simulink model "EMJ1"  (R2022b)
settings: Solver=VariableStepAuto  StartTime=0.0  StopTime=sim_time  FixedStep=0.001  RelTol=1e-3
values from neighbouring files (symbols this model uses):
  alpha = 0    [PMS.m]
  B = 0.24    [PMS.m]
  i = i:0.05:(i+0.5)    [PMS.m]
  Kb = 0.35    [PMS.m]
  Kt = 0.9    [PMS.m]
  L = 2.5  * (10^-3)    (= 0.0025)    [PMS.m]
  R = 0.03    [PMS.m]
  r = 0.3    [PMS.m]
  slope = 1    [PMS.m]
  v = 0    [PMS.m]
  velocity = 1    [PMS.m]
  W = 45    [PMS.m]
  X = 0.46    [PMS.m]
  Y = 300    [PMS.m]
  Z = 3000    [PMS.m]
libraries: simulink x1
settings Model: Creator=Gebruiker  LastModifiedBy=Gebruiker
settings SolverCC: MaxConsecutiveMinStep=2
settings DataIOCC: ReturnWorkspaceOutputs=off
settings ModelReferenceCC: EnableRefExpFcnMdlSchedulingChecks=on

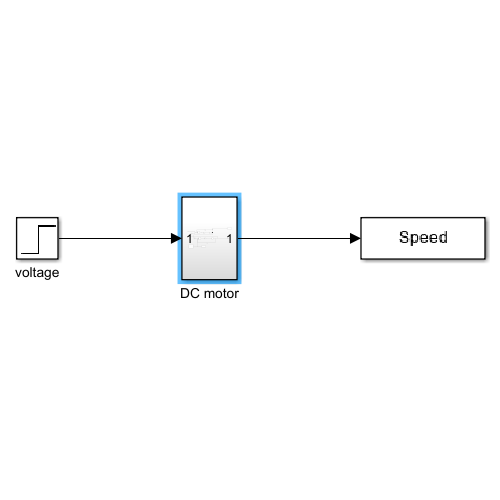
[thumbnail: Simulink's stored preview of the top-level diagram]
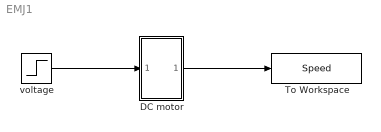
== system EMJ1 ==
  DC motor : Subsystem
  To Workspace : ToWorkspace  VariableName=Speed  SampleTime=-1
  voltage : Step  Time=0.1  After=48  SampleTime=0
  wires:
  DC motor/1(Out1) -> To Workspace/1
  voltage/1 -> DC motor/1(In1)

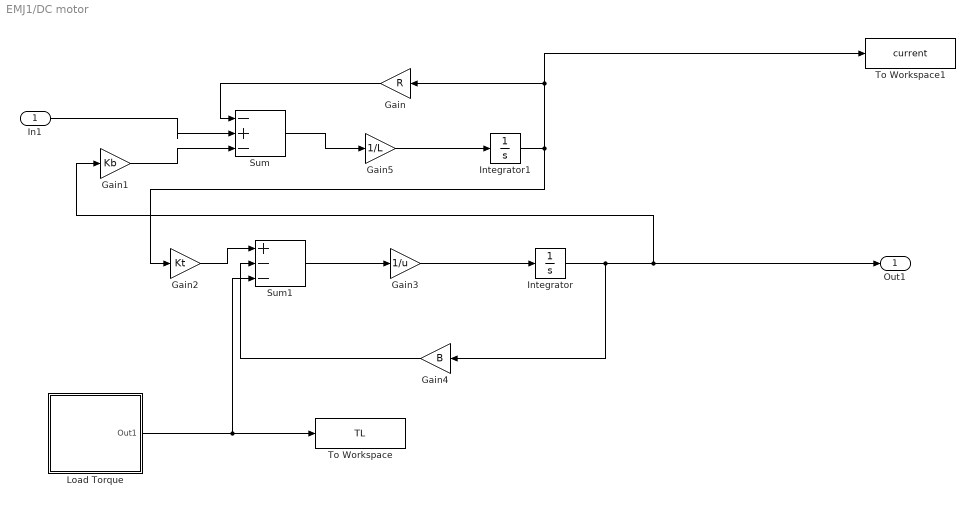
== system EMJ1/DC motor ==
  In1 : Inport
  Gain : Gain  Gain=R
  Gain1 : Gain  Gain=Kb
  Gain2 : Gain  Gain=Kt
  Gain3 : Gain  Gain=1/u
  Gain4 : Gain  Gain=B
  Gain5 : Gain  Gain=1/L
  Integrator : Integrator
  Integrator1 : Integrator
  Load Torque : Subsystem
  Sum : Sum  Inputs=|-+-
  Sum1 : Sum  Inputs=|+--
  To Workspace : ToWorkspace  VariableName=TL  SaveFormat=Timeseries  SampleTime=-1
  To Workspace1 : ToWorkspace  VariableName=current  SampleTime=-1
  Out1 : Outport
  wires:
  In1/1 -> Sum/2
  Gain/1 -> Sum/1
  Gain1/1 -> Sum/3
  Gain2/1 -> Sum1/1
  Sum1/1 -> Gain3/1
  Gain3/1 -> Integrator/1
  Sum/1 -> Gain5/1
  Gain5/1 -> Integrator1/1
  Gain4/1 -> Sum1/2
  Integrator1/1 -> Gain2/1, To Workspace1/1, Gain/1
  Integrator/1 -> Gain4/1, Out1/1, Gain1/1
  Load Torque/1(Out1) -> Sum1/3, To Workspace/1

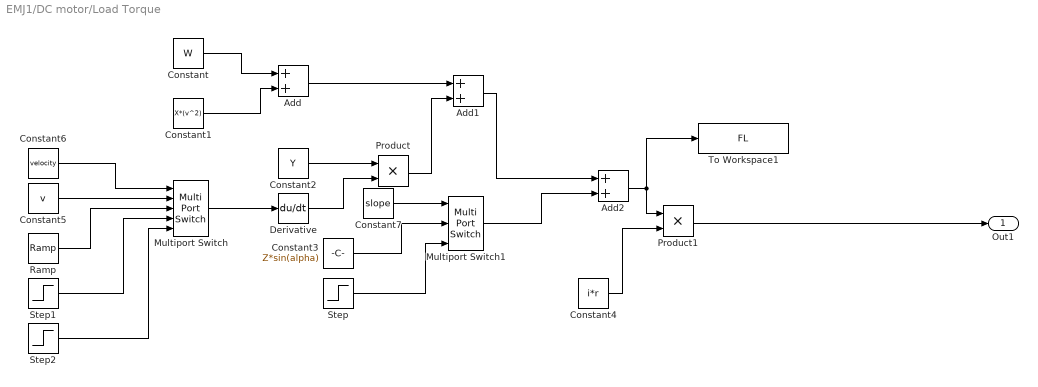
== system EMJ1/DC motor/Load Torque ==
  Add : Sum
  Add1 : Sum
  Add2 : Sum
  Constant : Constant  Value=W
  Constant1 : Constant  Value=X*(v^2)
  Constant2 : Constant  Value=Y
  Constant3 : Constant  Value=Z*sin(alpha)
  Constant4 : Constant  Value=i*r
  Constant5 : Constant  Value=v
  Constant6 : Constant  Value=velocity
  Constant7 : Constant  Value=slope
  Derivative : Derivative
  Multiport Switch : MultiPortSwitch  Inputs=4  SaturateOnIntegerOverflow=off  InputSameDT=off
  Multiport Switch1 : MultiPortSwitch  Inputs=2  SaturateOnIntegerOverflow=off  InputSameDT=off
  Product : Product
  Product1 : Product
  Ramp : simulink/Sources/Ramp  slope=10/0.5  start=0.5  InitialOutput=0
  Step : Step  Time=0.5  After=3  SampleTime=0
  Step1 : Step  After=10  SampleTime=0
  Step2 : Step  Time=0.001  After=4  SampleTime=0
  To Workspace1 : ToWorkspace  VariableName=FL  SampleTime=-1
  Out1 : Outport
  wires:
  Add2/1 -> To Workspace1/1, Product1/1
  Constant1/1 -> Add/2
  Add1/1 -> Add2/1
  Add/1 -> Add1/1
  Derivative/1 -> Product/2
  Constant4/1 -> Product1/2
  Constant/1 -> Add/1
  Product/1 -> Add1/2
  Constant2/1 -> Product/1
  Multiport Switch/1 -> Derivative/1
  Constant6/1 -> Multiport Switch/1
  Constant5/1 -> Multiport Switch/2
  Multiport Switch1/1 -> Add2/2
  Constant3/1 -> Multiport Switch1/2
  Step/1 -> Multiport Switch1/3
  Constant7/1 -> Multiport Switch1/1
  Step1/1 -> Multiport Switch/4
  Ramp/1 -> Multiport Switch/3
  Step2/1 -> Multiport Switch/5
  Product1/1 -> Out1/1
